simulink model "test_com_SensorFusion_SF_D4"  (R2019b)
settings: Solver=FixedStepDiscrete  StartTime=0  StopTime=stop  FixedStep=0.001  RelTol=1e-3
undefined symbols (not defined in the file or in its folder): BxTM, ByTM, CxTM, CyTM, g, gamma_stat_front, gamma_stat_rear, gearbox_ratio, l_F, l_R, m_sprung, m_unsprung_quarter, mag_calib_front_center, mag_calib_front_compmatrix, mag_calib_rear_center, mag_calib_rear_compmatrix, should_be_in_theSensorFusion, switch_VelYcalculation_pSF, testStart_VelX_pSF, testVelY_pSF, tire_r_dyn, track_angle_front, track_width_front, track_width_rear, v2o_x, wheel_kinematics_breakpoints, wheel_kinematics_FL_data, wheel_kinematics_FR_data, wheelbase, x9DFrontX, x9DFrontY, x9DRearX, x9DRearY
libraries: SignalProcessingSensorFusionLib x30, simulink x6
(part 4 of 9)

== matlab function test_com_SensorFusion_SF_D4/Subsystem14/SensorFusion_E9/kalman ==
  data: x9DFront input; x9DRear input; VehicleState output Bus: control_VehicleState size=1; bias output single size=18; state output single size=20; Covariance output single; v2o input; WheelSpeeds input; WheelSpeeds_Sq input; RockerAngle input; RockerAngle_Sq input; dt input; x9DFrontX parameter; x9DRearX parameter; v2o_x parameter; track_width_front parameter; track_width_rear parameter; z_output output single; avarageWSpeed output; m_sprung parameter; m_unsprung_quarter parameter; J_Sxx parameter; J_Syy parameter; l_R parameter; l_F parameter; wheelbase parameter; h_aero parameter; rho_air parameter; h_cg parameter; cdA parameter; clA_front parameter; clA_rear parameter; motion_ratio_front parameter; motion_ratio_rear parameter; motion_ratio_heave_front parameter; motion_ratio_heave_rear parameter; motion_ratio_roll_front parameter; motion_ratio_roll_rear parameter; spring_stiff_heave_front parameter; spring_stiff_heave_rear parameter; damp_coef_heave_front_push parameter size=[1 3]; damp_coef_heave_front_pull parameter size=[1 3]; damp_coef_heave_rear_push parameter size=[1 3]; damp_coef_heave_rear_pull parameter size=[1 3]; spring_stiff_roll_front parameter; spring_stiff_roll_rear parameter; damp_coef_roll_front_push parameter size=[1 3]; damp_coef_roll_front_pull parameter size=[1 3]; damp_coef_roll_rear_push parameter size=[1 3]; damp_coef_roll_rear_pull parameter size=[1 3]; x_hat_tl output single; y_tl output single; g parameter; tire_r_dyn parameter; mag_calib_front_compmatrix parameter; mag_calib_rear_compmatrix parameter; mag_calib_rear_center parameter; mag_calib_front_center input; delta input; Output output
function [VehicleState, bias, state, Covariance, z_output , avarageWSpeed, x_hat_tl, y_tl, Output] ...
    = kalman(x9DFront, x9DRear, v2o, WheelSpeeds, WheelSpeeds_Sq, RockerAngle, RockerAngle_Sq,...
    dt, x9DFrontX, x9DRearX, v2o_x, track_width_front, track_width_rear, ...
    m_sprung,  m_unsprung_quarter, J_Sxx, J_Syy, l_R, l_F, wheelbase, h_aero, rho_air, h_cg, cdA, clA_front, clA_rear,...
    motion_ratio_front, motion_ratio_rear, ...
    motion_ratio_heave_front, motion_ratio_heave_rear, motion_ratio_roll_front, motion_ratio_roll_rear, ...
    spring_stiff_heave_front, spring_stiff_heave_rear, ...
    damp_coef_heave_front_push, damp_coef_heave_front_pull, damp_coef_heave_rear_push, damp_coef_heave_rear_pull,...
    spring_stiff_roll_front, spring_stiff_roll_rear, ...
    damp_coef_roll_front_push, damp_coef_roll_front_pull, damp_coef_roll_rear_push, damp_coef_roll_rear_pull, ...
    g, tire_r_dyn,...
    mag_calib_front_compmatrix, mag_calib_rear_compmatrix, mag_calib_rear_center, ...
mag_calib_front_center, delta)

persistent x bias_x P bias_P k  
persistent slipangle_zero_counter no_slipanglesensor_counter slipanglesensor_counter
persistent i time_count bias_counter
persistent WheelSpeedsCloseTogether_counter WheelSpeedsNoJump_counter
persistent WheelSpeeds_old yawRate_old rollAng_old pitchAng_old PosZ_old v2o_VelX_old
persistent Heading_Front_old Heading_Rear_old magnetoffset

%%


%motion_ratio_front= 0.00045;
%motion_ratio_rear= 0.0013;
%motion_ratio_heave_front= 1.178;
%motion_ratio_heave_rear= 0.5795;
%motion_ratio_roll_front= 1.674;
%motion_ratio_roll_rear= 0.408;
%% Setup

% kalman filter
% x_k+1 = F x_k + w_k
% z_k = H x_k + v_k

% State vector
% x = [
%       VelX;            % (1)   Velocity in x-direction
%       VelY;           % (2)   Velocity in y-direction
%       PosZ;           % (3)   position of the car in z-direction
%       VelZ;           % (4)   velocity of the car in y-direction
%       AccX;           % (5)   Acceleration in x-direction of the car (CG)
%       AccY;           % (6)        -"-        y-direction  
%       AccZ;           % (7)   Acceleration in z-direction of the car (CG)
%       RollAng;        % (8)   RollAngle of the Monocoque
%       RollRate;       % (9)   RollRate of the Monocoque
%       RollAcc;        % (10)  RollAcceleration of the Monocoque 
%       PitchAng;       % (11)  PitchAngle of the Monocoque
%       PitchRate;      % (12)  PitchRate of the Monocoque
%       PitchAcc;       % (13)  PitchAcceleration of the Monocoque 
%       YawAng;         % (14)   YawAngle of the Monocoque
%       YawRate;        % (15)   YawRate of the Monocoque
%       YawAcc;         % (16)  YawAcceleration of the Monocoque 
%       RockerAngFL;    % (17)  Rocker Angle of front left rocker
%       RockerAngFR;    % (18)  Rocker Angle of front left rocker
%       RockerAngHL;    % (19)  Rocker Angle of front left rocker
%       RockerAngHR;    % (20)  Rocker Angle of front left rocker

% Bias State vector
% bias_x = [
%       b_x_a1;         % (1)   Bias 1. acceleration sensor in x-direction Front
%       b_y_a1;         % (2)                -"-               y-direction Front
%       b_z_a1;         % (3)                -"-               z-direction Front
%       b_x_a2;         % (4)   Bias 2. acceleration sensor in x-direction Rear 
%       b_y_a2;         % (5)                -"-               y-direction Rear
%       b_z_a2;         % (6)                -"-               z-direction Rear
%       b_rollRate1;    % (7)   Bias 1. gyroscope around z-axis
%       b_pitchRate1;   % (8)   Bias 1. gyroscope around z-axis
%       b_yawRate1;     % (9)   Bias 1. gyroscope around z-axis
%       b_rollRate2;    % (10)  Bias 2. gyroscope around z-axis
%       b_pitchRate2;   % (11)  Bias 2. gyroscope around z-axis
%       b_yawRate2;    % (12)  Bias 2. gyroscope around z-axis
%       b_RockerAngFL;  % (13)  Rocker Angle of front left rocker
%       b_RockerAngFR;  % (14)  Rocker Angle of front left rocker
%       b_RockerAngHL;  % (15)  Rocker Angle of front left rocker
%       b_RockerAngHR;  % (16)  Rocker Angle of front left rocker
%       LateralIntegratorError]; %(17) Error is made during the inegration
%       LongitudinalIntegratorError]; %(18) Error is made during the inegration

num_states=20;
num_bias_states=18;

% sample time dt [seconds]
% THE SAMPLE TIME DOESN'T HAVE TO BE GIVEN MANUALLY ANYMORE, BECAUSE
% CURRENTLY IT'S GIVEN AS AN INPUT FROM THE SIMULINK SUBSYSTEMS SAMPLE TIME
% dt=0.001; 

if isempty(P)
    %init
    % Transformation  (normative matrix * (measured signal - offset))
    CompCorrFront = mag_calib_front_compmatrix * ([x9DFront.MagX; x9DFront.MagY; x9DFront.MagZ] - mag_calib_front_center);
    CompCorrRear = mag_calib_rear_compmatrix * ([x9DRear.MagX; x9DRear.MagY; x9DRear.MagZ] - mag_calib_rear_center);

    % Yaw angle calculation based on normalized magnetic compass data
    Heading_Front_old = -1*atan2(CompCorrFront(2,:), CompCorrFront(1,:)); % intervall [0,2*pi];
    Heading_Rear_old = -1*atan2(CompCorrRear(2,:), CompCorrRear(1,:)); % intervall [0,2*pi];

    Heading_Front_old = -Heading_Front_old;
    Heading_Rear_old = -Heading_Rear_old;
    magnetoffset = Heading_Rear_old - Heading_Front_old;
    
    i=1;
    time_count=1;
    bias_counter=1;
    
    slipangle_zero_counter=single(0);
    no_slipanglesensor_counter=0;
    slipanglesensor_counter=0;
    
    WheelSpeedsCloseTogether_counter=0;
    WheelSpeedsNoJump_counter=0;
    
    k = 1;
    
    x = single(zeros(num_states,1));
    P = single(zeros(num_states, num_states));
    
    bias_x = single(zeros(num_bias_states,1));
    bias_P = single(zeros(num_bias_states, num_bias_states)); 
    
    yawRate_old=single(0); % this value is for the derivation of the yaw rate 
    WheelSpeeds_old=single([0;0;0;0]);
    rollAng_old=single([0;0]);
    pitchAng_old=single([0;0]);
    PosZ_old=single([0;0]);
    v2o_VelX_old=single(0);
end



%% Transformation of 9D-Magnetfield to Yaw-Angle

% Transformation  (normative matrix * (measured signal - offset))
CompCorrFront = mag_calib_front_compmatrix * ([x9DFront.MagX; x9DFront.MagY; x9DFront.MagZ] - mag_calib_front_center);
CompCorrRear = mag_calib_rear_compmatrix * ([x9DRear.MagX; x9DRear.MagY; x9DRear.MagZ] - mag_calib_rear_center);

% Yaw angle calculation based on normalized magnetic compass data


HeadingFront = -1*atan2(CompCorrFront(2,:), CompCorrFront(1,:)) + magnetoffset; % intervall [0,2*pi];
HeadingRear = -1*atan2(CompCorrRear(2,:), CompCorrRear(1,:)); % intervall [0,2*pi];


HeadingFront = -HeadingFront;
HeadingRear = -HeadingRear;

if(Heading_Front_old-HeadingFront < -pi)
HeadingFront = HeadingFront - round(abs(Heading_Front_old-HeadingFront)/(2*pi))*2*pi;
elseif(Heading_Front_old-HeadingFront > pi)
HeadingFront = HeadingFront + round(abs(Heading_Front_old-HeadingFront)/(2*pi))*2*pi;
end

if(Heading_Rear_old-HeadingRear < -pi)
HeadingRear = HeadingRear - round(abs(Heading_Rear_old-HeadingRear)/(2*pi))*2*pi;
elseif(Heading_Rear_old-HeadingRear > pi)
HeadingRear = HeadingRear + round(abs(Heading_Rear_old-HeadingRear)/(2*pi))*2*pi;
end


Heading_Front_old = HeadingFront;
Heading_Rear_old = HeadingRear;


%% Preparing WheelSpeeds

% Differenz durchschnittl. Raddrehzahl / Schwimmwinkelsensor > Schwellwert
% -> Schwimmwinkelsensor nicht vertrauen

WheelSpeeds = WheelSpeeds * tire_r_dyn; % dynamischer Reifenradius


% Durchschnittliche Raddrehzahl ermitteln
avgWheelSpeed = mean(WheelSpeeds);
%(WheelSpeeds.WheelSpeed_FL + WheelSpeeds.WheelSpeed_FR + WheelSpeeds.WheelSpeed_RL + WheelSpeeds.WheelSpeed_RR) / 4;
avarageWSpeed=single(avgWheelSpeed);

WheelDistances = [-track_width_front/2; track_width_front/2; ...
    -track_width_rear/2; track_width_rear/2];
WheelSpeeds_at_CoG=WheelSpeeds+WheelDistances*x(15);

MinWheelSpeed = min(WheelSpeeds_at_CoG);
MaxWheelSpeed = max(WheelSpeeds_at_CoG);


if((max(abs(WheelSpeeds-WheelSpeeds_old))/dt)<10)
    WheelSpeedsNoJump_counter=WheelSpeedsNoJump_counter+1;
else
    WheelSpeedsNoJump_counter=0;
end
if(MaxWheelSpeed-avgWheelSpeed<0.6 && avgWheelSpeed-MinWheelSpeed<0.6)
    WheelSpeedsCloseTogether_counter=WheelSpeedsCloseTogether_counter+1;
else
    WheelSpeedsCloseTogether_counter=0;
end


%% valueIsNew Slipangle Sensor
valueIsNew = false;
if(v2o_VelX_old~=v2o.VelX)
    valueIsNew = true;
    v2o_VelX_old=v2o.VelX;
end

%% Preparation TireLoad

% MonoShock Auswahl Druck/Zug-Stufe
if -x(12)*l_F + x(4) > 0  %Vorne Druck
    damp_coef_heave_front = damp_coef_heave_front_push;
else                    %Vorne Zug
    damp_coef_heave_front = damp_coef_heave_front_pull;
end

if x(12)*l_R + x(4) > 0  %Hinten Druck
    damp_coef_heave_rear = damp_coef_heave_rear_push;
else                    %Hinten Zug
    damp_coef_heave_rear = damp_coef_heave_rear_pull;
end


% Rolldämpfer Auswahl Druck/Zug-Stufe
if x(9) < 0             % if Bedingung muss überprüft werden!
    damp_coef_roll_front = damp_coef_roll_front_push;
    damp_coef_roll_rear = damp_coef_roll_rear_push;
else
    damp_coef_roll_front = damp_coef_roll_front_pull;
    damp_coef_roll_rear = damp_coef_roll_rear_pull; 
end
damp_F=@(v,damp_coef)(v*0.5*(damp_coef(2)+damp_coef(3))+sign(v)*(0.5*(damp_coef(2)-damp_coef(3))*(damp_coef(1)-abs(v*sign(v)-damp_coef(1)))));


%% Prediction 

measure_bias=false;
if(avgWheelSpeed < 0.01 )
    if bias_counter*dt>1 && bias_counter*dt<9
        measure_bias=true;
    end
else % update the state only if the biases are currently not measured
    
    % nonlinear system-equotations
    x=[
        %       VelX;            % (1)   Velocity in x-direction
        x(1)+dt*(x(5)+x(2)*x(15));
        %       VelY;           % (2)   Velocity in y-direction
        x(2)+dt*(x(6)-x(1)*x(15)); %x_2+dt*((x_6/x_1)-x_15)
        %       PosZ;           % (3)   position of the car in z-direction
        x(3);
        %       VelZ;           % (4)   velocity of the car in y-direction
        x(4);
        %       AccX;           % (5)   Acceleration in x-direction of the car (CG)
        x(5);
        %       AccY;           % (6)        -"-        y-direction  
        x(6);
        %       AccZ;           % (7)   Acceleration in x-direction of the car (CG)
        x(7);
        %       RollAng;        % (8)   RollAngle of the Monocoque
        x(8);
        %       RollRate;       % (9)   RollRate of the Monocoque
        x(9);
        %       RollAcc;        % (10)  RollAcceleration of the Monocoque
        x(10);
        %       PitchAng;       % (11)  PitchAngle of the Monocoque
        x(11);
        %       PitchRate;      % (12)  PitchRate of the Monocoque
        x(12)+dt*x(13);
        %       PitchAcc;       % (13)  PitchAcceleration of the Monocoque 
        x(13);
        %       YawAng;         % (14)   YawAngle of the Monocoque
        x(14)+dt*x(15);
        %       YawRate;        % (15)   YawRate of the Monocoque
        x(15);
        %       YawAcc;         % (16)  YawAcceleration of the Monocoque 
        x(16);
        %       RockerAngFL;    % (17)  Rocker Angle of front left rocker
        x(17);
        %       RockerAngFR;    % (18)  Rocker Angle of front left rocker
        x(18);
        %       RockerAngHL;    % (19)  Rocker Angle of front left rocker
        x(19);
        %       RockerAngHR;    % (20)  Rocker Angle of front left rocker
        x(20);
        ];

    %Calculating a linearized A Matrix
    A=[ %                                                           1                                                       2                   3               4                       5                           6    7            8             9    10         11          12   13  14            15  16  17  18  19  20
                                                                        1,                                               dt*x(15),                  0,             0,                     dt,                           0,  0,           0,             0,  0,           0,          0,  0,  0,     dt*x(2),  0,  0,  0,  0,  0;
                                                                -x(15)*dt,                                                      1,                  0,             0,                      0,                          dt,  0,           0,             0,  0,           0,          0,  0,  0,  -(dt*x(1)),  0,  0,  0,  0,  0;
                                                                        0,                                                      0,                  1,             0,                      0,                           0,  0,           0,             0,  0,           0,          0,  0,  0,           0,  0,  0,  0,  0,  0;
                                                                        0,                                                      0,                  0,             1,                      0,                           0,  0,           0,             0,  0,           0,          0,  0,  0,           0,  0,  0,  0,  0,  0;
                                                                        0,                                                      0,                  0,             0,                      1,                           0,  0,           0,             0,  0,           0,          0,  0,  0,           0,  0,  0,  0,  0,  0;
                                                                        0,                                                      0,                  0,             0,                      0,                           1,  0,           0,             0,  0,           0,          0,  0,  0,           0,  0,  0,  0,  0,  0;
                                                                        0,                                                      0,                  0,             0,                      0,                           0,  1,           0,             0,  0,           0,          0,  0,  0,           0,  0,  0,  0,  0,  0;
                                                                        0,                                                      0,                  0,             0,                      0,                           0,  0,           1,             0,  0,           0,          0,  0,  0,           0,  0,  0,  0,  0,  0;
                                                                        0,                                                      0,                  0,             0,                      0,                           0,  0,           0,             0,  0,           0,          0,  0,  0,           0,  0,  0,  0,  0,  0;
                                                                        0,                                                      0,                  0,             0,                      0,                           0,  0,           0,             0,  1,           0,          0,  0,  0,           0,  0,  0,  0,  0,  0;
                                                                        0,                                                      0,                  0,             0,                      0,                           0,  0,           0,             0,  0,           1,          0,  0,  0,           0,  0,  0,  0,  0,  0;
                                                                        0,                                                      0,                  0,             0,                      0,                           0,  0,           0,             0,  0,           0,          1, dt,  0,           0,  0,  0,  0,  0,  0;
                                                                        0,                                                      0,                  0,             0,                      0,                           0,  0,           0,             0,  0,           0,          0,  1,  0,           0,  0,  0,  0,  0,  0;
                                                                        0,                                                      0,                  0,             0,                      0,                           0,  0,           0,             0,  0,           0,          0,  0,  1,          dt,  0,  0,  0,  0,  0;
                                                                        0,                                                      0,                  0,             0,                      0,                           0,  0,           0,             0,  0,           0,          0,  0,  0,           1,  0,  0,  0,  0,  0;
                                                                        0,                                                      0,                  0,             0,                      0,                           0,  0,           0,             0,  0,           0,          0,  0,  0,           0,  1,  0,  0,  0,  0;
                                                                        0,                                                      0,                  0,             0,                      0,                           0,  0,           0,             0,  0,           0,          0,  0,  0,           0,  0,  1,  0,  0,  0;
                                                                        0,                                                      0,                  0,             0,                      0,                           0,  0,           0,             0,  0,           0,          0,  0,  0,           0,  0,  0,  1,  0,  0;
                                                                        0,                                                      0,                  0,             0,                      0,                           0,  0,           0,             0,  0,           0,          0,  0,  0,           0,  0,  0,  0,  1,  0;
                                                                        0,                                                      0,                  0,             0,                      0,                           0,  0,           0,             0,  0,           0,          0,  0,  0,           0,  0,  0,  0,  0,  1;];


    %A = dt*F + eye(length(F));

    W = eye(num_states);

    exp=single(0.4/((0.2*(x(5)-1)^2)+1)-2.4);%(0.4*(2^(-0.1*(x(5)-1)^2))-3.1);%-2.7*2^(-0.1*(x(5)-1)^2)-3.1*(-2^(-0.1*(x(5)-1)^2)+1) % This exponent is a value between -2.1 (if x(5)=2) and -4.5 (if x(5) is away from 2)
    % Covariance matrix of state noise
    Q = diag( ...     
            [10^exp %VelX;       % (1)   Velocity in x
            1;       %       Velocity in y;      % (2)   Velocity in y
            0.0001;        %       PosZ;           % (3)   position of the car in z-direction
            0.0001;        %       VelZ;           % (4)   velocity of the car in y-direction
            0.0005;      %       AccX;           % (5)   Acceleration in x-direction of the car (CG)
            0.0005;       %       AccY;           % (6)        -"-        y-direction  
            0.00001;       %       AccZ;           % (7)   Acceleration in x-direction of the car (CG)
            0.00001;        %       RollAng;        % (8)   RollAngle of the Monocoque
            0.0001;      %       RollRate;       % (9)   RollRate of the Monocoque
            0.0002;       %       RollAcc;        % (10)  RollAcceleration of the Monocoque 
            0.00001;        %       PitchAng;       % (11)  PitchAngle of the Monocoque
            0.0001;      %       PitchRate;      % (12)  PitchRate of the Monocoque
            0.0002;       %       PitchAcc;       % (13)  PitchAcceleration of the Monocoque 
            0.05;       %       YawAng;         % (14)   YawAngle of the Monocoque
            0.00001;      %       YawRate;        % (15)   YawRate of the Monocoque
            0.001;       %       YawAcc;         % (16)  YawAcceleration of the Monocoque 
            0.00001;       %       RockerAngFL;    % (17)  Rocker Angle of front left rocker
            0.00001;       %       RockerAngFR;    % (18)  Rocker Angle of front left rocker
            0.00001;       %       RockerAngHL;    % (19)  Rocker Angle of front left rocker
            0.00001;  ...  %       RockerAngHR;    % (20)  Rocker Angle of front left rocker
            ]*0.002);

    % prediction calculation
    %x = x + dt*F*x; % + dt*B*u;          % statevector update
    %NO LINEAR EQUOTATION USED, THEREFORE ONLY THE LINEARIZED MATRIX A IS USED
    %TO UPDATE P

    P = A*P*A' + W*Q*W';                 % covariance matrix update
    bias_counter=0;
end 

bias_P = bias_P+eye(num_bias_states)*0.00000001;

%% calculating turning Radius of car for Pfuschlösung if all 9D  or slipanglesensor
   if (abs(delta)>pi/180)
    r_y=single((wheelbase-x(1)*0.03+0.0)*tan(sign(delta)*(pi*0.5)-0.2047*3.76*delta));
   else
     r_y=single(9999999);
   end

%% Measurement SF

% Measurement selection: With the help of the singal qualifiers it is
% determined which signal can be used as a measurement input for the kalman
% filter
bias_selection=[];
selection=[18];
if (v2o.VelX_Sq<4) && (v2o.VelY_Sq<4) && abs(v2o.VelX-v2o_VelX_old) < 2
    slipanglesensor_counter=slipanglesensor_counter+1;
    no_slipanglesensor_counter=0;
end
if no_slipanglesensor_counter>5
    slipanglesensor_counter=0;
end
VelY_measurement=single(0);
if slipanglesensor_counter>5 && valueIsNew
    selection=[14 15 selection];
    VelY_measurement=v2o.VelY-x(15)*v2o_x ; 
else
    %if(WheelSpeedsNoJump_counter>7 && WheelSpeedsCloseTogether_counter>7 && abs(x(5))<10)
        
        %bias_selection=[bias_selection 18];
        selection=[selection 15 20 21 22];
   % end
   
    VelY_measurement=single(x(1)*(l_R-x(1)*0.03+0.0)/(r_y));
    no_slipanglesensor_counter=no_slipanglesensor_counter+1;
end

if (x9DFront.AccX_Sq<4)
    selection=[1 selection];
end

if (x9DFront.AccY_Sq<4)
    selection=[2 selection];
end

if (x9DRear.AccX_Sq<4)
    selection=[3 selection];
end

if (x9DRear.AccY_Sq<4)
    selection=[4 selection];
end

AccZ_Front=single(0);
AccZ_Rear=single(0);
if (x9DFront.AccZ_Sq<4)&&(x9DRear.AccZ_Sq<4)
    selection=[7 17 selection];
    AccZ_Front=x9DFront.AccZ;
    AccZ_Rear=x9DRear.AccZ;
end
if (x9DFront.AccZ_Sq<4)&&(x9DRear.AccZ_Sq>3)
    selection=[7 selection];
    AccZ_Front=x9DFront.AccZ;
    AccZ_Rear=x9DFront.AccZ;
end
if (x9DFront.AccZ_Sq>3)&&(x9DRear.AccZ_Sq<4)
    selection=[7 selection];
    AccZ_Front=x9DRear.AccZ;
    AccZ_Rear=x9DRear.AccZ;
end

if (x9DFront.AccY_Sq<4)&&(x9DRear.AccY_Sq<4)
    selection=[19 selection];
end

if (x9DFront.RollRate_Sq<4)
    selection=[8 selection];
end

if (x9DRear.RollRate_Sq<4)
    selection=[9 selection];
end

if (x9DFront.PitchRate_Sq<4)
    selection=[10 selection];
end

if (x9DRear.PitchRate_Sq<4)
    selection=[11 selection];
end

if (x9DFront.YawRate_Sq<4)
    selection=[12 selection];
end

if (x9DRear.YawRate_Sq<4)
    selection=[13 selection];
end

if (x9DRear.YawRate_Sq>3)&&(x9DFront.YawRate_Sq>3)%wenn beide 9D ausfallen pfuschlösung einschalten
    selection=[selection 30];
end
if (RockerAngle_Sq(1)<4)
	selection=[selection 23];
end

if (RockerAngle_Sq(2)<4)
	selection=[selection 24];
end

if (RockerAngle_Sq(3)<4)
	selection=[selection 25];
end

if (RockerAngle_Sq(4)<4)
	selection=[selection 26];
end

if ((RockerAngle_Sq(1)>3)&&(RockerAngle_Sq(2)>3)&&(RockerAngle_Sq(4)<4)&&(RockerAngle_Sq(3)<4))||((RockerAngle_Sq(3)>3)&&(RockerAngle_Sq(4)>3)&&(RockerAngle_Sq(1)<4)&&(RockerAngle_Sq(2)<4))
    delta_h=h_cg*x(5)*(m_sprung)/(2*(l_F*motion_ratio_heave_front^2*spring_stiff_heave_front+l_R*motion_ratio_heave_rear^2*spring_stiff_heave_rear));
    if((RockerAngle_Sq(1)>3)) %wenn die vorderen beiden FDS sensoren ausgefallen sind
        RH_RL=(RockerAngle(3)-bias_x(15))*motion_ratio_rear;                                                                      % (25)   pitch-angle (left)
        RH_RR=(RockerAngle(4)-bias_x(16))*motion_ratio_rear;
        RH_FL=RH_RL-delta_h;
        RH_FR=RH_RR-delta_h;
        selection=[selection 23 24];
    else
        RH_FL=(RockerAngle(1)-bias_x(13))*motion_ratio_front;                                                                     % (23)   roll-angle (front)
        RH_FR=(RockerAngle(2)-bias_x(14))*motion_ratio_front;
        RH_RL=RH_FL+delta_h;
        RH_RR=RH_FR+delta_h;
        selection=[selection 25 26];
    end
    
    
else
    RH_FL=(RockerAngle(1)-bias_x(13))*motion_ratio_front;                                                                     % (23)   roll-angle (front)
     RH_FR=(RockerAngle(2)-bias_x(14))*motion_ratio_front;                                                                     % (24)   roll-angle (rear)
     RH_RL=(RockerAngle(3)-bias_x(15))*motion_ratio_rear;                                                                      % (25)   pitch-angle (left)
     RH_RR=(RockerAngle(4)-bias_x(16))*motion_ratio_rear;  
end
selection=[5 6 selection 27 28 29];


if measure_bias==true
	bias_selection=1:16;
	selection=[16 20];
end


%zero slipangle while driving straight ahead
straightAheadBounds=single(0.1);
straightAheadDelayTimeSteps=25;
if(abs(x(15))<straightAheadBounds)
    slipangle_zero_counter=slipangle_zero_counter+((straightAheadBounds-abs(x(15)))^2)/((straightAheadBounds)^2);
    selection = [selection 16];
else
    
    slipangle_zero_counter=single(0);
end
if(slipangle_zero_counter>straightAheadDelayTimeSteps)
    
    slipangle_zero_counter=single(0);
end


% 1 only slip angle sensor (slip angle)
% 2 only front 9D sensor (9D sensor)
% 3 only rear 9D sensor (9D sensor)
% 4 one 9D sensor missing (slip angle + (front) 9D sensor)
% 5 one 9D sensor missing (slip angle + (rear) 9D sensor)
% 6 long time no slip angle sensor (use motor revs for speed measurement)
% 7 no slip angle sensor (2 * 9D sensor)
% 8 all sensors available(slip angle + 2 * 9D sensors)
% 0 no sensors except wheeel speeds

%%



AccZ_CoG=((AccZ_Front-bias_x(3))*abs(x9DFrontX)+(AccZ_Rear-bias_x(6))*abs(x9DRearX))/(abs(x9DFrontX) +abs(x9DRearX));

if (x9DFront.AccX_Sq<4)||(x9DRear.AccX_Sq<4)
    AccX_CoG=((x9DFront.AccX+x9DRear.AccX-bias_x(1)-bias_x(4))/2.0)-AccZ_CoG*x(11);
    accx_meas_precision=0.0001;
else
    AccX_CoG=(avgWheelSpeed-mean(WheelSpeeds_old))/dt;
    accx_meas_precision=0.002;
end
WheelSpeeds_old=WheelSpeeds;


if (x9DFront.AccY_Sq<4)||(x9DRear.AccY_Sq<4)
    AccY_CoG=((x9DFront.AccY-bias_x(2))*abs(x9DFrontX)+(x9DRear.AccY-bias_x(5))*abs(x9DRearX))/(abs(x9DFrontX) +abs(x9DRearX))+AccZ_CoG*x(8);
else
    AccY_CoG=(x(1)^2)/r_y;
end
%AccZ_CoG=(x9DFront.AccZ*abs(x9DRearX)+x9DRear.AccZ*abs(x9DFrontX))/(abs(x9DFrontX) +abs(x9DRearX));
% Measured states
    
z1 = [
     x9DFront.AccX-bias_x(1)-(AccZ_Front-bias_x(3))*x(11); %- x(6)^2*x9DFrontX;                       % (1)   x-Acc (front)
     (x9DFront.AccY-bias_x(2))+(AccZ_Front-bias_x(3))*x(8); %                                            % (2)   y-Acc (front)
     x9DRear.AccX-bias_x(4)-(AccZ_Rear-bias_x(6))*x(11); %- x(6)^2*x9DRearX ;                         % (3)   x-Acc (rear)
     (x9DRear.AccY-bias_x(5))+(AccZ_Rear-bias_x(6))*x(8);                                                % (4)   y-Acc (rear)
     AccX_CoG;                                                                            % (5)   x-Acc (average)
     AccY_CoG;                                                                                % (6)   y-Acc (average)
     AccZ_CoG;                                                                                              % (7)   z-Acc (average)
     x9DFront.RollRate-bias_x(7);                                                                           % (8)   roll-rate (front)
     x9DRear.RollRate-bias_x(10);                                                                           % (9)   roll-rate (rear)
     x9DFront.PitchRate-bias_x(8);                                                                          % (10)   pitch-rate (front)
     x9DRear.PitchRate-bias_x(11);                                                                          % (11)   pitch-rate (rear)
     x9DFront.YawRate-bias_x(9);                                                                            % (12)   yaw-rate (front)
     x9DRear.YawRate-bias_x(12);                                                                            % (13)   yaw-rate (rear)
     v2o.VelX;                                                             % (14)   velocity x
     VelY_measurement;                                                                                         % (15)    velocity y
     0 ;                                                                                                    % (16)     velocity y zeroing
     (AccZ_Front-bias_x(3)-(AccZ_Rear-bias_x(6)))/(abs(x9DFrontX) +abs(x9DRearX));                    % (17)  pitch-acceleration
     (x(15)-yawRate_old)/dt;                                                                                % (18)  yaw-acceleration Front (derivation of yaw Rate)
     (x9DFront.AccY - x9DRear.AccY-bias_x(2)+bias_x(5))/(abs(x9DFrontX) +abs(x9DRearX)) ;                   % (19)  yaw-acceleration
     avgWheelSpeed;                                                                                         % (20) average wheelspeed
     MinWheelSpeed;                                                                     % (21) wheelspeed of slowest wheel
     MaxWheelSpeed;                                                                     % (22) wheelspeed of fastest wheel
     RH_FL;                                                                     % (23)   roll-angle (front)
     RH_FR;                                                                     % (24)   roll-angle (rear)
     RH_RL;                                                                      % (25)   pitch-angle (left)
     RH_RR;                                                                      % (26)   pitch-angle (right)
     (x(8)-rollAng_old(2))/(2*dt);                                                                          % (27)   rollRate (derivate of roll Angle)
     (x(11)-pitchAng_old(2))/(2*dt);                                                                        % (28)   pitchRate (derivate of pitch Angle)
     (x(3)-PosZ_old(2))/(dt*2);                                                                             % (29) z-velocity (dervitate of posZ)
     x(1)/r_y;                                                                                          % (30)   z-position as mean of the wheel-travels of 3 wheels (FL,FR,HR)
     0;                                                                                           % (31)   z-position as mean of the wheel-travels of 3 wheels (FL,FR,HL)
    ];
  
yawRate_old=x(15); % Save old yawRate to calculate the yawAcc by derivation
rollAng_old(2)=rollAng_old(1);
rollAng_old(1)=x(8);
pitchAng_old(2)=pitchAng_old(1);
pitchAng_old(1)=x(11);
PosZ_old(2)=PosZ_old(1);
PosZ_old(1)=x(3);

kill_matrix=zeros(length(z1),length(z1));
z=single(zeros(size(z1)));
for w=1:length(selection)
    z(selection(w))=z1(selection(w));    
    kill_matrix(selection(w),selection(w))=1.0;
end

% Measurement function with "selection" vector considered (only use the measurements which are new and correct)
h1 = [
     x(5)-x9DFrontX*x(15)^2;     % (1)   x-Acc (front)
     x(6)+x9DFrontX*x(16);       % (2)   y-Acc (front)
     x(5)-x9DRearX*x(15)^2;      % (3)   x-Acc (rear)
     x(6)+x9DRearX*x(16);        % (4)   y-Acc (rear)
     x(5);                       % (5)   x-Acc (average)
     x(6);                       % (6)   y-Acc (average)
     x(7);                       % (7)   z-Acc (average)   
     x(9) ;                      % (8)   roll-rate (front)
     x(9) ;                      % (9)   roll-rate (rear)
     x(12) ;                     % (10)  pitch-rate (front)
     x(12) ;                     % (11)  pitch-rate (rear)
     x(15) ;                     % (12)  yaw-rate (front)
     x(15) ;                     % (13)  yaw-rate (rear)
     x(1);% - x(15)*v2oY*0;      % (14)  velocity
     x(2);%+;                    % (15)  slip-angle
     x(2);%+;                    % (16)  slip-angle zeroing
     x(13);                      % (17)  pitch-acceleration
     x(16);                      % (18)  yaw-acceleration (dervation of yawRate)
     x(16);                      % (19)  yaw-acceleration
     x(1);             % (20)  average wheelspeed
     x(1);             % (21)  wheelspeed of slowest
     x(1);             % (22)  wheelspeed of fastest
     x(3)-track_width_front*0.5*x(8)-l_F*x(11); % (23)   wheel lift FL 
     x(3)+track_width_front*0.5*x(8)-l_F*x(11); % (24)   wheel lift FR 
     x(3)-track_width_rear*0.5*x(8)+l_R*x(11);  % (25)   wheel lift RL
     x(3)+track_width_rear*0.5*x(8)+l_R*x(11);  % (26)   wheel lift RR
     x(9) ;                      % (27)   roll Rate (derivate of roll angle)
     x(12) ;                     % (28)   pitch Rate (derivate of pitch angle)
     x(4) ;                      % (29)   z velocity (derivate of Z Pos )
     x(15);                      % (30)   yaw-rate from pfusch über dynamischer drehungsradius;
     0;                      % (31)   Heading Yaw-Angle Rear
     ];
     
h=kill_matrix*h1;

%Calculate linearized measurement matrix H

H1=[ %      1     2   3     4   5     6     7                    8     9    10    11  12  13  14  15   16  17  18  19  20
            0 ,   0 , 0 ,   0 , 1 ,   0 ,   0 ,                  0 ,   0 ,   0 ,   0 , 0 , 0 , 0 , 0 ,  0 , 0 , 0 , 0 , 0 ;         %1
            0 ,   0 , 0 ,   0 , 0 ,   1 ,   0 ,                  0 ,   0 ,   0 ,   0 , 0 , 0 , 0 , 0 ,  0 , 0 , 0 , 0 , 0 ;         %2
            0 ,   0 , 0 ,   0 , 1 ,   0 ,   0 ,                  0 ,   0 ,   0 ,   0 , 0 , 0 , 0 , 0 ,  0 , 0 , 0 , 0 , 0 ;     %3
            0 ,   0 , 0 ,   0 , 0 ,   1 ,   0 ,                  0 ,   0 ,   0 ,   0 , 0 , 0 , 0 , 0 ,  0 , 0 , 0 , 0 , 0 ;     %4
            0 ,   0 , 0 ,   0 , 1 ,   0 ,   0 ,                  0 ,   0 ,   0 ,   0 , 0 , 0 , 0 , 0 ,  0 , 0 , 0 , 0 , 0 ;     %5
            0 ,   0 , 0 ,   0 , 0 ,   1 ,   0 ,                  0 ,   0 ,   0 ,   0 , 0 , 0 , 0 , 0 ,  0 , 0 , 0 , 0 , 0 ;     %6
            0 ,   0 , 0 ,   0 , 0 ,   0 ,   1 ,                  0 ,   0 ,   0 ,   0 , 0 , 0 , 0 , 0 ,  0 , 0 , 0 , 0 , 0 ;     %7
            0 ,   0 , 0 ,   0 , 0 ,   0 ,   0 ,                  0 ,   1 ,   0 ,   0 , 0 , 0 , 0 , 0 ,  0 , 0 , 0 , 0 , 0 ;     %8
            0 ,   0 , 0 ,   0 , 0 ,   0 ,   0 ,                  0 ,   1 ,   0 ,   0 , 0 , 0 , 0 , 0 ,  0 , 0 , 0 , 0 , 0 ;     %9
            0 ,   0 , 0 ,   0 , 0 ,   0 ,   0 ,                  0 ,   0 ,   0 ,   0 , 1 , 0 , 0 , 0 ,  0 , 0 , 0 , 0 , 0 ;     %10
            0 ,   0 , 0 ,   0 , 0 ,   0 ,   0 ,                  0 ,   0 ,   0 ,   0 , 1 , 0 , 0 , 0 ,  0 , 0 , 0 , 0 , 0 ;     %11
            0 ,   0 , 0 ,   0 , 0 ,   0 ,   0 ,                  0 ,   0 ,   0 ,   0 , 0 , 0 , 0 , 1 ,  0 , 0 , 0 , 0 , 0 ;     %12
            0 ,   0 , 0 ,   0 , 0 ,   0 ,   0 ,                  0 ,   0 ,   0 ,   0 , 0 , 0 , 0 , 1 ,  0 , 0 , 0 , 0 , 0 ;     %13
            1 ,   0 , 0 ,   0 , 0 ,   0 ,   0 ,                  0 ,   0 ,   0 ,   0 , 0 , 0 , 0 , 0 ,  0 , 0 , 0 , 0 , 0 ;     %14
            0 ,   1 , 0 ,   0 , 0 ,   0 ,   0 ,                  0 ,   0 ,   0 ,   0 , 0 , 0 , 0 , 0 ,  0 , 0 , 0 , 0 , 0 ;     %15
            0 ,   1 , 0 ,   0 , 0 ,   0 ,   0 ,                  0 ,   0 ,   0 ,   0 , 0 , 0 , 0 , 0 ,  0 , 0 , 0 , 0 , 0 ;     %16
            0 ,   0 , 0 ,   0 , 0 ,   0 ,   0 ,                  0 ,   0 ,   0 ,   0 , 0 , 1 , 0 , 0 ,  0 , 0 , 0 , 0 , 0 ;     %17
            0 ,   0 , 0 ,   0 , 0 ,   0 ,   0 ,                  0 ,   0 ,   0 ,   0 , 0 , 0 , 0 , 0 ,  1 , 0 , 0 , 0 , 0 ;     %18
            0 ,   0 , 0 ,   0 , 0 ,   0 ,   0 ,                  0 ,   0 ,   0 ,   0 , 0 , 0 , 0 , 0 ,  1 , 0 , 0 , 0 , 0 ;     %19
            1 ,   0 , 0 ,   0 , 0 ,   0 ,   0 ,                  0 ,   0 ,   0 ,   0 , 0 , 0 , 0 , 0 ,  0 , 0 , 0 , 0 , 0 ;     %20
            1 ,   0 , 0 ,   0 , 0 ,   0 ,   0 ,                  0 ,   0 ,   0 ,   0 , 0 , 0 , 0 , 0 ,  0 , 0 , 0 , 0 , 0 ;     %21    
            1 ,   0 , 0 ,   0 , 0 ,   0 ,   0 ,                  0 ,   0 ,   0 ,   0 , 0 , 0 , 0 , 0 ,  0 , 0 , 0 , 0 , 0 ;     %22
            0 ,   0 , 1 ,   0 , 0 ,   0 ,   0 ,-track_width_front*0.5,   0 ,   0 , -l_F, 0 , 0 , 0 , 0 ,  0 , 0 , 0 , 0 , 0 ;     %23
            0 ,   0 , 1 ,   0 , 0 ,   0 ,   0 , track_width_front*0.5,   0 ,   0 , -l_F, 0 , 0 , 0 , 0 ,  0 , 0 , 0 , 0 , 0 ;     %24
            0 ,   0 , 1 ,   0 , 0 ,   0 ,   0 , -track_width_rear*0.5,   0 ,   0 ,  l_R, 0 , 0 , 0 , 0 ,  0 , 0 , 0 , 0 , 0 ;     %25
            0 ,   0 , 1 ,   0 , 0 ,   0 ,   0 ,  track_width_rear*0.5,   0 ,   0 ,  l_R, 0 , 0 , 0 , 0 ,  0 , 0 , 0 , 0 , 0 ;    %26
            0 ,   0 , 0 ,   0 , 0 ,   0 ,   0 ,                  0 ,   1 ,   0 ,   0 , 0 , 0 , 0 , 0 ,  0 , 0 , 0 , 0 , 0 ;     %27
            0 ,   0 , 0 ,   0 , 0 ,   0 ,   0 ,                  0 ,   0 ,   0 ,   0 , 1 , 0 , 0 , 0 ,  0 , 0 , 0 , 0 , 0 ;    %28
            0 ,   0 , 0 ,   1 , 0 ,   0 ,   0 ,                  0 ,   0 ,   0 ,   0 , 0 , 0 , 0 , 0 ,  0 , 0 , 0 , 0 , 0 ;    %29
            0 ,   0 , 0 ,   0 , 0 ,   0 ,   0 ,                  0 ,   0 ,   0 ,   0 , 0 , 0 , 0 , 1 ,  0 , 0 , 0 , 0 , 0 ;     %30
            0 ,   0 , 0 ,   0 , 0 ,   0 ,   0 ,                  0 ,   0 ,   0 ,   0 , 0 , 0 , 0 , 0 ,  0 , 0 , 0 , 0 , 0 ];    %31
H=kill_matrix*H1; 

factor=(1-(1/(WheelSpeedsNoJump_counter+1)))*(1-(1/(WheelSpeedsCloseTogether_counter+1)));%(1-(2^(-WheelSpeedsNoJump_counter)))*(1-(2^(-WheelSpeedsCloseTogether_counter)));
exp1=-2.4/(0.5*(x(5))^2+1)*factor-5*10^(-x(1));%-2.4*2^(-0.3*(x(5))^2)*factor-3*10^(-x(1));

exp2=-1.4/(0.5*(x(5)-5)^2+1)*factor;%-1.4*2^(-0.3*(x(5)-5)^2)*factor;

exp3=-2/(0.4*(x(5)+5)^2+1)*factor;%-2*2^(-0.2*(x(5)+5)^2)*factor;

div=(10-(9/(slipanglesensor_counter*0.01+1)));

R = diag([     
    0.001;                       % (1)   x-Acc (front)
    0.001;                       % (2)   y-Acc (front)
    0.001;                       % (3)   x-Acc (rear)
    0.001;                       % (4)   y-Acc (rear)
    accx_meas_precision;                       % (5)   x-Acc (average)
    0.0001;                       % (6)   y-Acc (average)
    0.0001;                       % (7)   z-Acc (average)
    0.1;                        % (8)   roll-rate (front)
    0.1;                        % (9)   roll-rate (rear)
    0.1;                        % (10)   pitch-rate (front)
    0.1;                        % (11)   pitch-rate (rear)
    0.0001;                     % (12)   yaw-rate (front)
    0.0001;                     % (13)   yaw-rate (rear)
    0.001/div;                     % (14)   velocity (from slip angle)
    0.01/div;                     % (15)   slipangle (beta)
    10^(-slipangle_zero_counter*3/(50.0));                       % (16)   slip-angle zeroing
    0.005;                      % (17)  pitch-acceleration
    0.005;                      % (18)  yaw-acceleration (derivation of yaw Rate)
    0.05;                       % (19)  yaw-acceleration
    10^exp1;                    % (20)  average speed of wheel
    10^exp2;                    % (21)  speed of slowest wheel
    10^exp3;                    % (22)  speed of fastest wheel
    0.001;                     % (23)   wheel lift FL
    0.001;                     % (24)   wheel lift FR
    0.001;                     % (25)   wheel lift RL
    0.001;                     % (26)   wheel lift RR
    0.00001;                     % (27)   roll Rate derivate of roll angle
    0.00001;                     % (28)   pitch Rate derivate of pitch angle
    0.001;                     % (29)   z velocity derivate of z-position
    0.001;                     % (30)   heading front (yaw Angle from magnetic field)
    0.00001                      % (31)   heading rear  (yaw Angle)
    ]);

bias_z1 =[
    x9DFront.AccX;      %       b_x_a1;         % (1)   Bias 1. acceleration sensor in x-direction Front
    x9DFront.AccY;      %       b_y_a1;         % (2)                -"-               y-direction Front
    x9DFront.AccZ+9.81; %       b_z_a1;         % (3)                -"-               z-direction Front
    x9DRear.AccX;       %       b_x_a2;         % (4)   Bias 2. acceleration sensor in x-direction Rear 
    x9DRear.AccY;       %       b_y_a2;         % (5)                -"-               y-direction Rear
    x9DRear.AccZ+9.81;  %       b_z_a2;         % (6)                -"-               z-direction Rear
    x9DFront.RollRate;  %       b_rollRate1;    % (7)   Bias 1. gyroscope around z-axis
    x9DFront.PitchRate; %       b_pitchRate1;   % (8)   Bias 1. gyroscope around z-axis
    x9DFront.YawRate;   %       b_yawRate1;     % (9)   Bias 1. gyroscope around z-axis
    x9DRear.RollRate;   %       b_rollRate2;    % (10)  Bias 2. gyroscope around z-axis
    x9DRear.PitchRate;  %       b_pitchRate2;   % (11)  Bias 2. gyroscope around z-axis
    x9DRear.YawRate;    %       b_yawRate2;     % (12)  Bias 2. gyroscope around z-axis
    RockerAngle(1);     %       b_RockerAngFL;  % (13)  Rocker Angle of front left rocker
    RockerAngle(2);     %       b_RockerAngFR;  % (14)  Rocker Angle of front left rocker
    RockerAngle(3);     %       b_RockerAngHL;  % (15)  Rocker Angle of front left rocker
    RockerAngle(4);     %       b_RockerAngHR]; % (16)  Rocker Angle of front left rocker
    0; %   LatIE           % (17)
    0; %   LongIE     % (18)  
    ];
 
bias_kill_matrix=zeros(length(bias_z1),length(bias_z1));
bias_z=single(zeros(size(bias_z1)));
for w=1:length(bias_selection)
    bias_z(bias_selection(w))=bias_z1(bias_selection(w));    
    bias_kill_matrix(bias_selection(w),bias_selection(w))=1.0;
end
bias_H=bias_kill_matrix*eye(num_bias_states);

bias_R = diag([ 
    0.001;    %       b_x_a1;         % (1)   Bias 1. acceleration sensor in x-direction Front
	0.001;    %       b_y_a1;         % (2)                -"-               y-direction Front
	0.001;    %       b_z_a1;         % (3)                -"-               z-direction Front
	0.001;    %       b_x_a2;         % (4)   Bias 2. acceleration sensor in x-direction Rear 
	0.001;    %       b_y_a2;         % (5)                -"-               y-direction Rear
	0.001;    %       b_z_a2;         % (6)                -"-               z-direction Rear
	0.001;    %       b_rollRate1;    % (7)   Bias 1. gyroscope around z-axis
	0.001;    %       b_pitchRate1;   % (8)   Bias 1. gyroscope around z-axis
	0.001;    %       b_yawRate1;     % (9)   Bias 1. gyroscope around z-axis
 	0.001;    %       b_rollRate2;    % (10)  Bias 2. gyroscope around z-axis
	0.001;    %       b_pitchRate2;   % (11)  Bias 2. gyroscope around z-axis
	0.001;    %       b_yawRate2;     % (12)  Bias 2. gyroscope around z-axis
	0.001;    %       b_RockerAngFL;  % (13)  Rocker Angle of front left rocker
	0.001;    %       b_RockerAngFR;  % (14)  Rocker Angle of front left rocker
	0.001;    %       b_RockerAngHL;  % (15)  Rocker Angle of front left rocker
	0.001;    %       b_RockerAngHR]; % (16)  Rocker Angle of front left rocker
    0.001;%10^(-2-(LateralIntegratorError_counter/5000));
    0.001;%10^(-2-(LateralIntegratorError_counter/5000));
    ]);


% Correction equations
I = eye(length(x));
V = eye(length(z));

K_tmp = P*H'/(H*P*H'+V*R*V');

x = x + K_tmp*(z-h);
P = (I - K_tmp*H)*P;


bias_K_tmp = bias_P*bias_H'/(bias_H*bias_P*bias_H'+bias_R);

bias_x = bias_x + bias_K_tmp*(bias_z-bias_H*bias_x);
bias_P = (eye(length(bias_x)) - bias_K_tmp*bias_H)*bias_P;

%% Check Vel
if x(1)<0
    x(1)=0;
end

%% Output 
VehicleState.PosX = single(0);
VehicleState.PosY = single(0);

VehicleState.VelX = x(1);
VehicleState.VelY = x(2);
VehicleState.YawAngle = x(14);
VehicleState.YawRate = x(15);
VehicleState.YawAcc = x(16);
VehicleState.AccX = x(5);
VehicleState.AccY = x(6);
VehicleState.AccZ = x(7);

z_output = z1;

state=x;
bias=bias_x;
Covariance = single(P);

k = k+1;

if(i==10000)
%     
%     testsumme;
%     testsumme2;
%     testsumme3;
i = 1;
end
i = i+1;
time_count=time_count+1;
bias_counter=bias_counter+1;

%% Output TireLoad
% Ausgang
Output=[x(3); x(4); x(8); x(9); x(11); x(12)];
%Nicht-Lineare Ausgangsmatrix
C_tl = [  (2*motion_ratio_heave_front^2*spring_stiff_heave_front*x(3)+ motion_ratio_heave_front*damp_F(2*motion_ratio_heave_front*x(4),damp_coef_heave_front)  -track_width_front*motion_ratio_roll_front^2*spring_stiff_roll_front*x(8)+  motion_ratio_roll_front*damp_F(-track_width_front*motion_ratio_roll_front*x(9),damp_coef_roll_front)  -2*l_F*motion_ratio_heave_front^2*spring_stiff_heave_front*x(11)+  motion_ratio_heave_front*damp_F(-2*l_F*motion_ratio_heave_front*x(12),damp_coef_heave_front));
          (2*motion_ratio_heave_front^2*spring_stiff_heave_front*x(3)+ motion_ratio_heave_front*damp_F(2*motion_ratio_heave_front*x(4),damp_coef_heave_front)+  track_width_front*motion_ratio_roll_front^2*spring_stiff_roll_front*x(8)+   motion_ratio_roll_front*damp_F(track_width_front*motion_ratio_roll_front*x(9),damp_coef_roll_front)  -2*l_F*motion_ratio_heave_front^2*spring_stiff_heave_front*x(11)+  motion_ratio_heave_front*damp_F(-2*l_F*motion_ratio_heave_front*x(12),damp_coef_heave_front));
            (2*motion_ratio_heave_rear^2*spring_stiff_heave_rear*x(3)+    motion_ratio_heave_rear*damp_F(2*motion_ratio_heave_rear*x(4),damp_coef_heave_rear)     -track_width_rear*motion_ratio_roll_rear^2*spring_stiff_roll_rear*x(8)+      motion_ratio_roll_rear*damp_F(-track_width_rear*motion_ratio_roll_rear*x(9),damp_coef_roll_rear)+    2*l_R*motion_ratio_heave_rear^2*spring_stiff_heave_rear*x(11)+      motion_ratio_heave_rear*damp_F(2*l_R*motion_ratio_heave_rear*x(12),damp_coef_heave_rear));
            (2*motion_ratio_heave_rear^2*spring_stiff_heave_rear*x(3)+    motion_ratio_heave_rear*damp_F(2*motion_ratio_heave_rear*x(4),damp_coef_heave_rear)+     track_width_rear*motion_ratio_roll_rear^2*spring_stiff_roll_rear*x(8)+       motion_ratio_roll_rear*damp_F(track_width_rear*motion_ratio_roll_rear*x(9),damp_coef_roll_rear)+    2*l_R*motion_ratio_heave_rear^2*spring_stiff_heave_rear*x(11)+      motion_ratio_heave_rear*damp_F(2*l_R*motion_ratio_heave_rear*x(12),damp_coef_heave_rear))];

D_tl = [m_unsprung_quarter + 0.5*m_sprung*l_R/wheelbase; 
        m_unsprung_quarter + 0.5*m_sprung*l_R/wheelbase; 
        m_unsprung_quarter + 0.5*m_sprung*l_F/wheelbase; 
        m_unsprung_quarter + 0.5*m_sprung*l_F/wheelbase]*g;

y_tl = C_tl  + D_tl;

% Begrenzung der Radlast
for n=1:1:4
    if y_tl(n) > 1800
        y_tl(n) = 1800;
    elseif y_tl(n) < 0
        y_tl(n) = 0;
    end
end

% Ausgabe
%os_z_tl     = - 0.5*(motion_ratio_front*x_tl(7)+motion_ratio_front*x_tl(8))*l_R/wheelbase - 0.5*(motion_ratio_rear*x_tl(9)+motion_ratio_rear*x_tl(10))*l_F/wheelbase;  
%os_phi_tl  = l_R/wheelbase*( x_tl(7)*motion_ratio_front - x_tl(8)*motion_ratio_front ) / track_width_front + l_F/wheelbase*( x_tl(9)*motion_ratio_rear - x_tl(10)*motion_ratio_rear ) / track_width_rear;
%os_theta_tl = ( motion_ratio_front*x_tl(7) + motion_ratio_front*x_tl(8) - motion_ratio_rear*x_tl(9) - motion_ratio_rear*x_tl(10) ) / 2 * wheelbase;

x_hat_tl  = [ x(3);
           x(4);
          (x(8))* 180 / pi;
           x(9)* 180 / pi;
          (x(11))* 180 / pi;
           x(12)* 180 / pi];



end
